simulink model "CameraAutomation"  (R2024a)
settings: Solver=FixedStepDiscrete  StartTime=0.0  StopTime=StopTime  FixedStep=0.1  RelTol=1e-3
libraries: VDriveToolbox x4
settings Model: Creator=tatsu  LastModifiedBy=ehsan
settings SolverCC: AlgebraicLoopSolver=TrustRegion
settings DebuggingCC: UnconnectedInputMsg=warning  UnconnectedOutputMsg=warning  UnconnectedLineMsg=warning
settings ModelReferenceCC: EnableRefExpFcnMdlSchedulingChecks=on
settings RTWCC: GPUComputeCapability=3.5

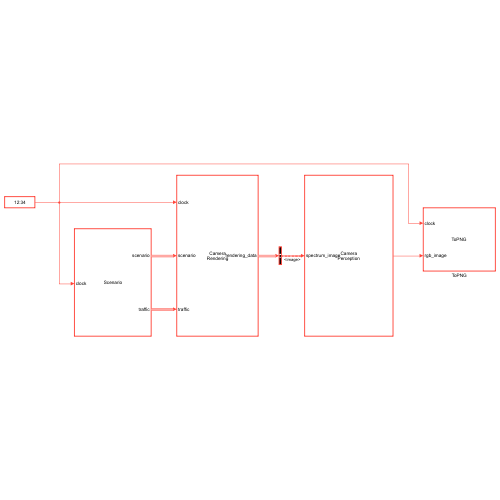
[thumbnail: Simulink's stored preview of the top-level diagram]
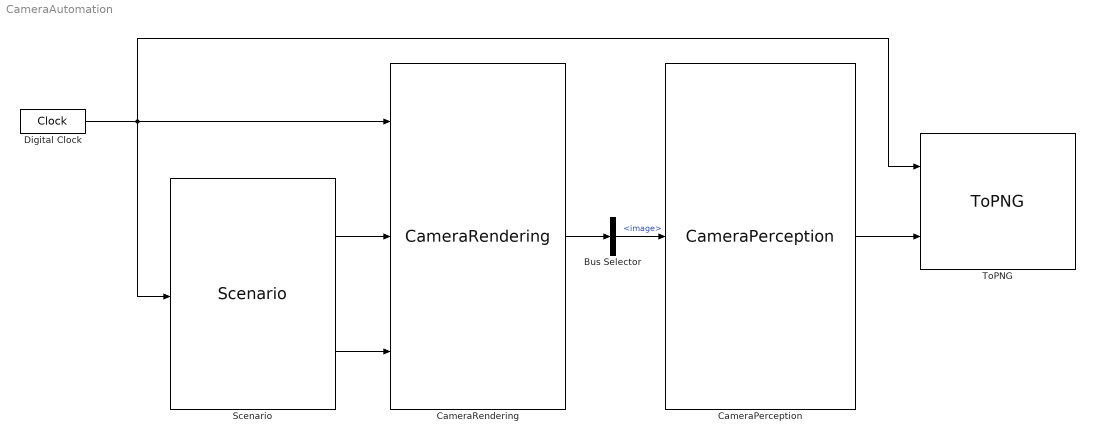
== system CameraAutomation ==
  Bus Selector : BusSelector  OutputSignals=image
  CameraPerception : VDriveToolbox/Cameras/CameraPerception  PerEControl=Manual  PerUBound=10.0  PerLBound=0.0  PerIsGamma="\"on\""
      settings: SourceProductName=V-Drive Toolbox
  CameraRendering : VDriveToolbox/Cameras/CameraRendering  SubConfigFile=cameraConfigFile  SubScenarioXML=scenarioXML  SubScenarioID=scenarioID  SubSensorID=sensorID  SubSampleTime=-1
      settings: SourceProductName=V-Drive Toolbox
  Digital Clock : DigitalClock  SampleTime=0.1
  Scenario : VDriveToolbox/Scenarios/Scenario  SubScenarioXML=scenarioXML  SubScenarioID=scenarioID
      settings: SourceProductName=V-Drive Toolbox
  ToPNG : VDriveToolbox/Cameras/ToPNG   file_name="\"image\""  dir=outputDir
      settings: SourceProductName=V-Drive Toolbox
  wires:
  Digital Clock/1 -> ToPNG/1, CameraRendering/1, Scenario/1
  Scenario/1 -> CameraRendering/2
  Scenario/2 -> CameraRendering/3
  CameraPerception/1 -> ToPNG/2
  CameraRendering/1 -> Bus Selector/1
  Bus Selector/1 -> CameraPerception/1  "<image>"
